simulink model "SimulinkLibrary"  (R2022b)
settings: Solver=VariableStepAuto  StartTime=0.0  StopTime=10.0  RelTol=1e-3
values from neighbouring files (symbols this model uses):
  A_w = [cosd(beta1)*sind(alfa1)  -cosd(beta2)*sind(alfa2) -cosd(beta3)*sind(alfa3) cosd(beta4)*sind(alfa4) ... (first row only)    [initfun_18072025.m]    (also in initfun_18072025_nogyro.m)
  A_wP = pinv(A_w)    [initfun_18072025.m]    (also in initfun_18072025_nogyro.m)
  C_d = 2.2    [initfun_18072025.m]    (also in initfun_18072025_nogyro.m)
  G_earth = 6.6742e-11    [initfun_18072025.m]    (also in initfun_18072025_nogyro.m)
  K = [F Z(:); Z(:)' sigma]    [Gain_matrix.m]    (also in QUEST.m = Gain_matrix(V',W',a); initfun_18072025.m = schmidt(nmax, mmax); initfun_18072025_nogyro.m = schmidt(nmax, mmax))
  m_earth = 5.9736e24    (= 5.9736e+24)    [initfun_18072025.m]    (also in initfun_18072025_nogyro.m)
  Magnetic_dipole = [0.1; 0.1;  0.1]    [initfun_18072025.m]    (also in initfun_18072025_nogyro.m)
  mmax = 3    [initfun_18072025.m]    (also in initfun_18072025_nogyro.m)
  nmax = 3    [initfun_18072025.m]    (also in initfun_18072025_nogyro.m)
  r_earth = 6371e3    (= 6371000)    [initfun_18072025.m]    (also in initfun_18072025_nogyro.m)
  RWs_Inertia = diag([9.0718e-06, 9.0718e-06, 9.0718e-06, 9.0718e-06])    [initfun_18072025.m]    (also in initfun_18072025_nogyro.m)
  RWs_Inertia_Inv = inv(RWs_Inertia)    [initfun_18072025.m]    (also in initfun_18072025_nogyro.m)
  Sat_Inertia = diag([6.295, 1.644, 5.462]*10^-1)    [initfun_18072025.m]    (also in initfun_18072025_nogyro.m)
undefined symbols (not defined in the file or in its folder): DiscIntNeverNeededParam, G, H, IAU, Sat_Aeromodel_det
libraries: matrix_library x4, vrlib x2, aerolibtransform2 x1
settings Model: Creator=LaMar  LastModifiedBy=LaMar

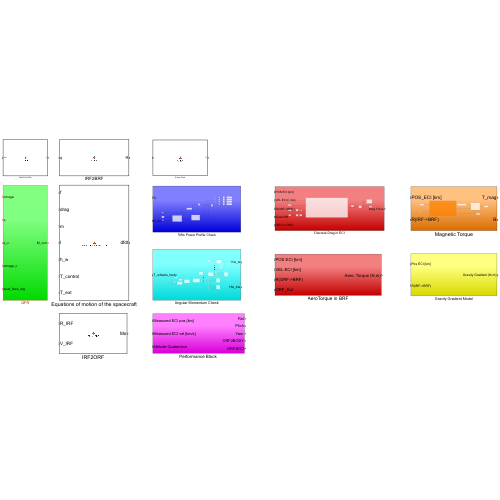
[thumbnail: Simulink's stored preview of the top-level diagram]
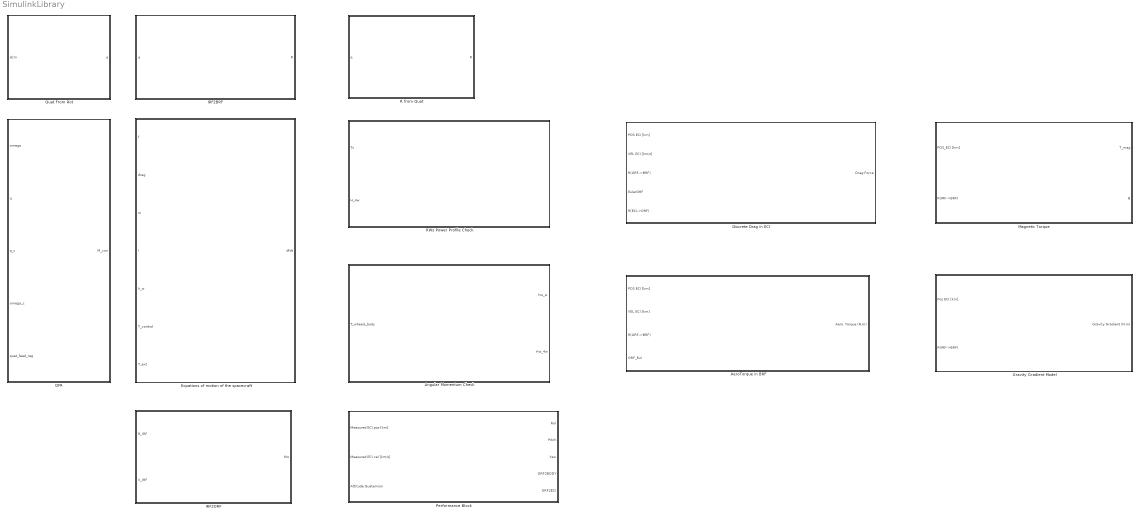
== system SimulinkLibrary ==
  AeroTorque in BRF : Subsystem
  Angular Momentum Check : Subsystem
  Discrete Drag in ECI : Subsystem
  Equations of motion of the spacecraft : MATLAB Function  TreatAsAtomicUnit=on
  Gravity Gradient Model : Subsystem
  IRF2BRF : MATLAB Function  TreatAsAtomicUnit=on
  IRF2ORF : MATLAB Function  TreatAsAtomicUnit=on
  Magnetic Torque : Subsystem
  "Performance Block " : Subsystem
  QFR : Subsystem
  Quat From Rot : MATLAB Function  TreatAsAtomicUnit=on
  R from Quat : MATLAB Function  TreatAsAtomicUnit=on
  RWs Power Profile Check : Subsystem

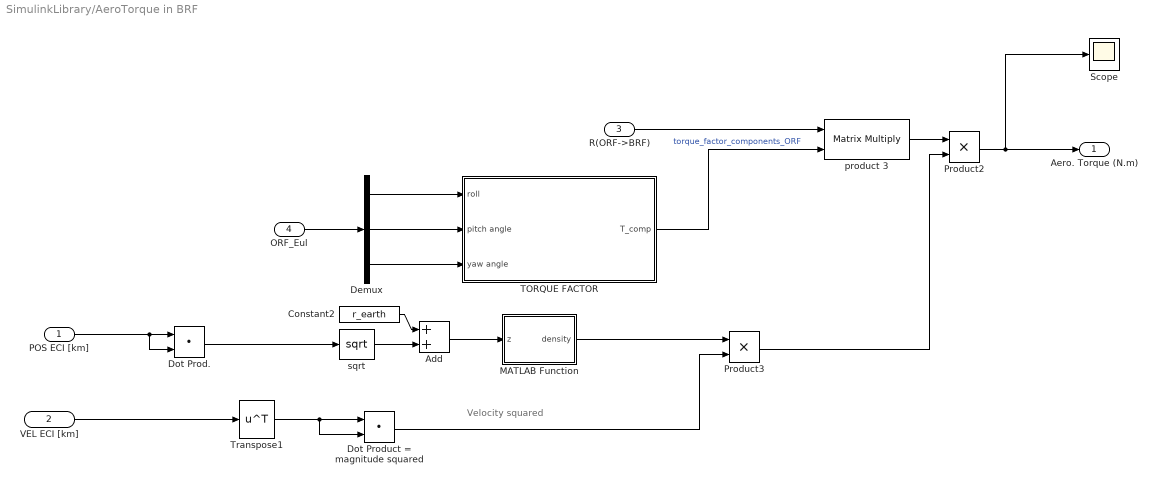
== system SimulinkLibrary/AeroTorque in BRF ==
  note: Velocity squared
  POS ECI [km] : Inport
  VEL ECI [km] : Inport  Port=2
  R(ORF->BRF) : Inport  Port=3
  ORF_Eul : Inport  Port=4
  Add : Sum
  Constant2 : Constant  Value=r_earth
  Demux : Demux  Outputs=3
  Dot Prod. : DotProduct  OutDataTypeStr=Inherit: Inherit via internal rule
  Dot Product = magnitude squared : DotProduct  OutDataTypeStr=Inherit: Inherit via internal rule
  MATLAB Function : MATLAB Function  TreatAsAtomicUnit=on
  Product2 : Product  RndMeth=Zero
  Product3 : Product  RndMeth=Zero
  Scope : Scope
  TORQUE FACTOR : Subsystem
  Transpose1 : Math  Operator=transpose  SignedPower=on
  product 3 : Product  Multiplication=Matrix(*)  RndMeth=Zero
  sqrt : Math  Operator=sqrt  SignedPower=on
  Aero. Torque (N.m) : Outport
  wires:
  sqrt/1 -> Add/2
  Add/1 -> MATLAB Function/1(z)
  Constant2/1 -> Add/1
  Demux/3 -> TORQUE FACTOR/3(yaw angle)
  Demux/2 -> TORQUE FACTOR/2(pitch angle)
  Demux/1 -> TORQUE FACTOR/1(roll)
  Product2/1 -> Aero. Torque (N.m)/1, Scope/1
  Dot Product = magnitude squared/1 -> Product3/2
  MATLAB Function/1(density) -> Product3/1
  VEL ECI [km]/1 -> Transpose1/1
  Transpose1/1 -> Dot Product = magnitude squared/1, Dot Product = magnitude squared/2
  TORQUE FACTOR/1(T_comp) -> product 3/2  "torque_factor_components_ORF"
  product 3/1 -> Product2/1
  Product3/1 -> Product2/2
  Dot Prod./1 -> sqrt/1
  POS ECI [km]/1 -> Dot Prod./2, Dot Prod./1
  R(ORF->BRF)/1 -> product 3/1
  ORF_Eul/1 -> Demux/1

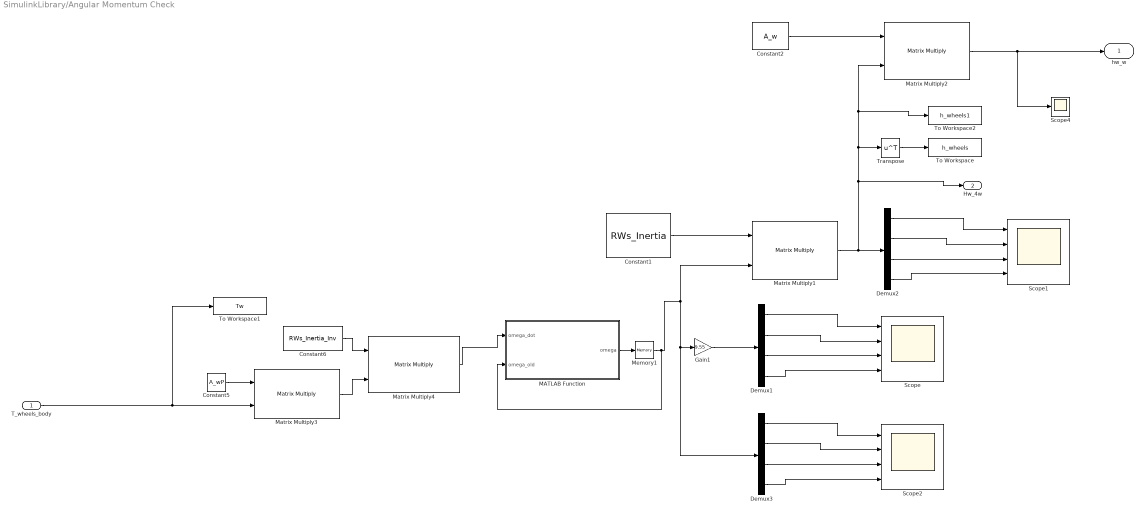
== system SimulinkLibrary/Angular Momentum Check ==
  T_wheels_body : Inport
  Constant1 : Constant  Value=RWs_Inertia
  Constant2 : Constant  Value=A_w
  Constant5 : Constant  Value=A_wP
  Constant6 : Constant  Value=RWs_Inertia_Inv
  Demux1 : Demux
  Demux2 : Demux
  Demux3 : Demux
  Gain1 : Gain  Gain=9.55
  MATLAB Function : MATLAB Function  TreatAsAtomicUnit=on
  Matrix Multiply{1..4} (4 alike) : Product  Multiplication=Matrix(*)
  Memory1 : Memory  InitialCondition=zeros(4,1)
  Scope : Scope  NumInputPorts=4
  Scope1 : Scope  NumInputPorts=4
  Scope2 : Scope  NumInputPorts=4
  Scope4 : Scope
  To Workspace : ToWorkspace  VariableName=h_wheels  SaveFormat=Structure  SampleTime=-1
      settings: Save2DSignal=2-D array (concatenate along first dimension)
  To Workspace1 : ToWorkspace  VariableName=Tw  SaveFormat=Structure With Time  SampleTime=-1
  To Workspace2 : ToWorkspace  VariableName=h_wheels1  SaveFormat=Structure  SampleTime=-1
      settings: Save2DSignal=2-D array (concatenate along first dimension)
  Transpose : Math  Operator=transpose
  hw_w : Outport
  Hw_4w : Outport  Port=2
  wires:
  Matrix Multiply1/1 -> Hw_4w/1, Transpose/1, To Workspace2/1, Matrix Multiply2/2, Demux2/1
  Constant2/1 -> Matrix Multiply2/1
  Demux1/4 -> Scope/4
  Matrix Multiply2/1 -> Scope4/1, hw_w/1
  Gain1/1 -> Demux1/1
  Demux1/3 -> Scope/3
  Demux1/2 -> Scope/2
  Demux1/1 -> Scope/1
  Constant5/1 -> Matrix Multiply3/1
  Constant1/1 -> Matrix Multiply1/1
  Demux2/3 -> Scope1/3
  Demux2/1 -> Scope1/1
  T_wheels_body/1 -> Matrix Multiply3/2, To Workspace1/1
  Demux2/4 -> Scope1/4
  Constant6/1 -> Matrix Multiply4/1
  Matrix Multiply3/1 -> Matrix Multiply4/2
  Demux2/2 -> Scope1/2
  Matrix Multiply4/1 -> MATLAB Function/1(omega_dot)
  MATLAB Function/1(omega) -> Memory1/1
  Demux3/3 -> Scope2/3
  Memory1/1 -> MATLAB Function/2(omega_old), Demux3/1, Gain1/1, Matrix Multiply1/2
  Demux3/2 -> Scope2/2
  Demux3/4 -> Scope2/4
  Demux3/1 -> Scope2/1
  Transpose/1 -> To Workspace/1

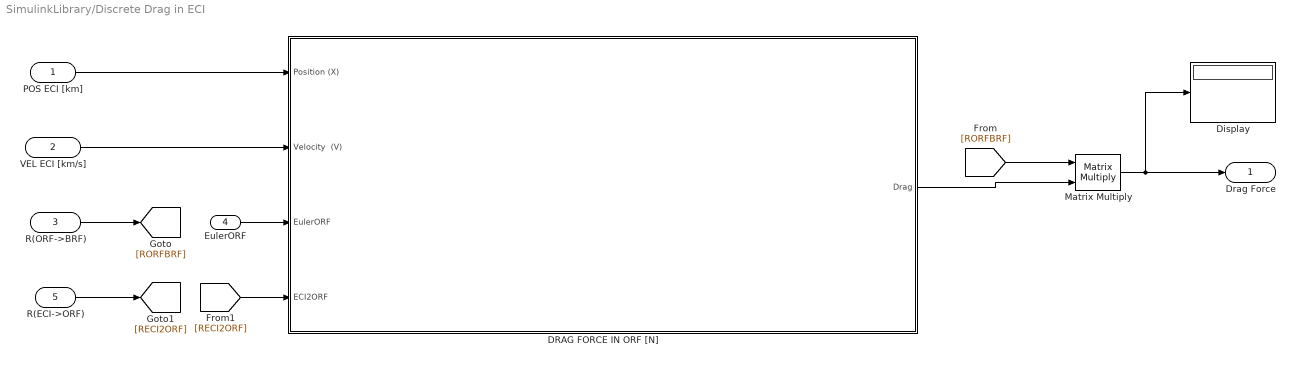
== system SimulinkLibrary/Discrete Drag in ECI ==
  POS ECI [km] : Inport
  VEL ECI [km/s] : Inport  Port=2
  R(ORF->BRF) : Inport  Port=3
  EulerORF : Inport  Port=4
  R(ECI->ORF) : Inport  Port=5
  DRAG FORCE IN ORF [N] : Subsystem
  Display : Display
  Matrix Multiply : Product  Multiplication=Matrix(*)
  Drag Force : Outport
  wires:
  R(ORF->BRF)/1 -> [RORFBRF]
  VEL ECI [km/s]/1 -> DRAG FORCE IN ORF [N]/2(Velocity  (V))
  POS ECI [km]/1 -> DRAG FORCE IN ORF [N]/1(Position (X))
  DRAG FORCE IN ORF [N]/1(Drag) -> Matrix Multiply/2
  Matrix Multiply/1 -> Display/1, Drag Force/1
  [RORFBRF] -> Matrix Multiply/1
  EulerORF/1 -> DRAG FORCE IN ORF [N]/3(EulerORF)
  [RECI2ORF] -> DRAG FORCE IN ORF [N]/4(ECI2ORF)
  R(ECI->ORF)/1 -> [RECI2ORF]

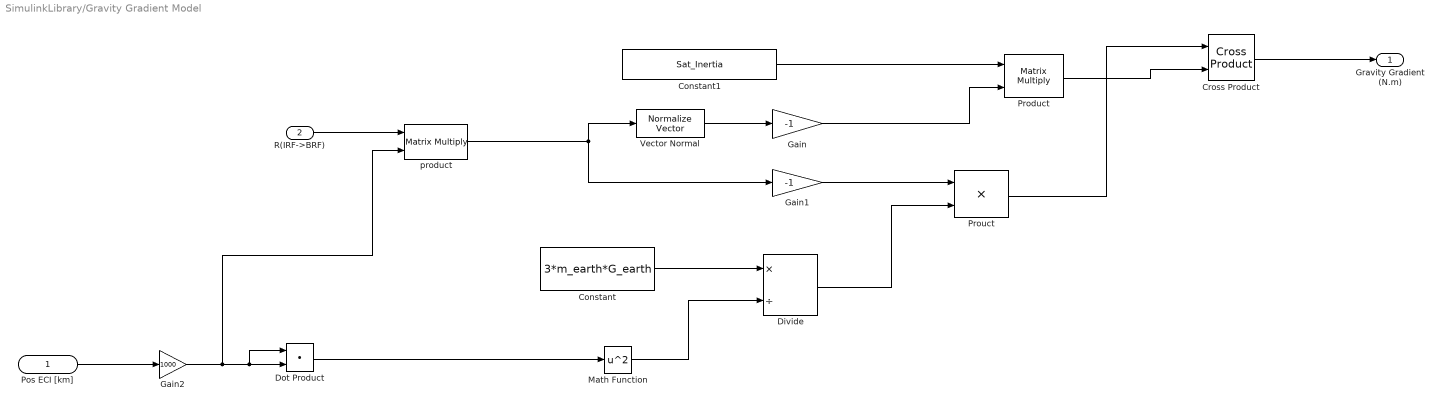
== system SimulinkLibrary/Gravity Gradient Model ==
  Pos ECI [km] : Inport
  R(IRF->BRF) : Inport  Port=2
  Constant : Constant  Value=3*m_earth*G_earth
  Constant1 : Constant  Value=Sat_Inertia
  Cross Product : matrix_library/Cross Product
  Divide : Product  Inputs=*/
  Dot Product : DotProduct  OutDataTypeStr=Inherit: Inherit via internal rule
  Gain : Gain  Gain=-1
  Gain1 : Gain  Gain=-1
  Gain2 : Gain  Gain=1000
  Math Function : Math  Operator=square  SignedPower=on
  Product : Product  Multiplication=Matrix(*)  RndMeth=Zero
  Prouct : Product  RndMeth=Zero
  Vector Normal : vrlib/Utilities/Normalize Vector  maxzero=0
  "product " : Product  Multiplication=Matrix(*)  RndMeth=Zero
  Gravity Gradient (N.m) : Outport
  wires:
  Divide/1 -> Prouct/2
  Constant/1 -> Divide/1
  Math Function/1 -> Divide/2
  Vector Normal/1 -> Gain/1
  Cross Product/1 -> Gravity Gradient (N.m)/1
  Dot Product/1 -> Math Function/1
  Product/1 -> Cross Product/2
  Constant1/1 -> Product/1
  "product "/1 -> Vector Normal/1, Gain1/1
  Gain1/1 -> Prouct/1
  Pos ECI [km]/1 -> Gain2/1
  Gain/1 -> Product/2
  Prouct/1 -> Cross Product/1
  R(IRF->BRF)/1 -> "product "/1
  Gain2/1 -> "product "/2, Dot Product/1, Dot Product/2

== system SimulinkLibrary/Magnetic Torque ==
  POS_ECI [km] : Inport
  R(IRF->BRF) : Inport  Port=2
  Cross Product : matrix_library/Cross Product
  Earth magnetc Field : Subsystem
  m : Constant  Value=Magnetic_dipole
  T_mag : Outport
  B : Outport  Port=2
  wires:
  POS_ECI [km]/1 -> Earth magnetc Field/1(R_ECI)
  Earth magnetc Field/1("BRF Earth magnetic field (T)  ") -> Cross Product/2, B/1
  m/1 -> Cross Product/1
  Cross Product/1 -> T_mag/1
  R(IRF->BRF)/1 -> Earth magnetc Field/2(R(IRF->BRF))

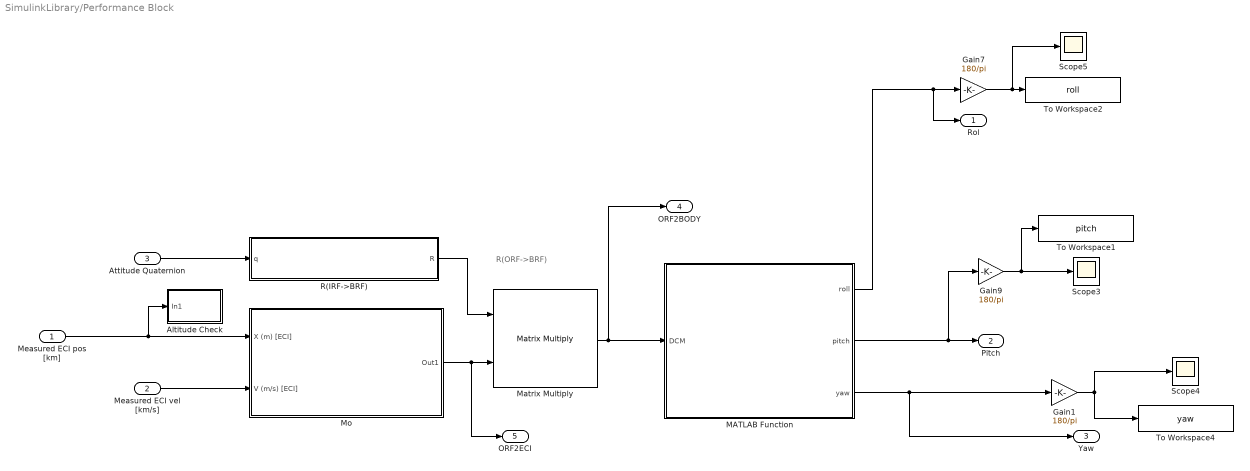
== system SimulinkLibrary/Performance Block  ==
  note: R(ORF->BRF)
  Measured ECI pos [km] : Inport
  Measured ECI vel [km/s] : Inport  Port=2
  "Attitude Quaternion " : Inport  Port=3
  Altitude Check : Subsystem
  Gain1 : Gain  Gain=180/pi
  Gain7 : Gain  Gain=180/pi
  Gain9 : Gain  Gain=180/pi
  MATLAB Function : MATLAB Function  TreatAsAtomicUnit=on
  Matrix Multiply : Product  Multiplication=Matrix(*)
  Mo : Subsystem
  R(IRF->BRF) : MATLAB Function  TreatAsAtomicUnit=on
  Scope3 : Scope
  Scope4 : Scope
  Scope5 : Scope
  To Workspace1 : ToWorkspace  VariableName=pitch  SaveFormat=Structure  SampleTime=-1
      settings: Save2DSignal=2-D array (concatenate along first dimension)
  To Workspace2 : ToWorkspace  VariableName=roll  SaveFormat=Structure  SampleTime=-1
      settings: Save2DSignal=2-D array (concatenate along first dimension)
  To Workspace4 : ToWorkspace  VariableName=yaw  SaveFormat=Structure  SampleTime=-1
      settings: Save2DSignal=2-D array (concatenate along first dimension)
  Rol : Outport
  Pitch : Outport  Port=2
  "Yaw " : Outport  Port=3
  ORF2BODY : Outport  Port=4
  ORF2ECI : Outport  Port=5
  wires:
  MATLAB Function/3(yaw) -> "Yaw "/1, Gain1/1
  MATLAB Function/1(roll) -> Gain7/1, Rol/1
  "Attitude Quaternion "/1 -> R(IRF->BRF)/1(q)
  Measured ECI vel [km/s]/1 -> Mo/2(V (m/s) [ECI])
  Gain1/1 -> Scope4/1, To Workspace4/1
  MATLAB Function/2(pitch) -> Pitch/1, Gain9/1
  Matrix Multiply/1 -> ORF2BODY/1, MATLAB Function/1(DCM)
  Gain7/1 -> To Workspace2/1, Scope5/1
  Mo/1(Out1) -> ORF2ECI/1, Matrix Multiply/2
  Gain9/1 -> To Workspace1/1, Scope3/1
  R(IRF->BRF)/1(R) -> Matrix Multiply/1
  Measured ECI pos [km]/1 -> Mo/1(X (m) [ECI]), Altitude Check/1(In1)

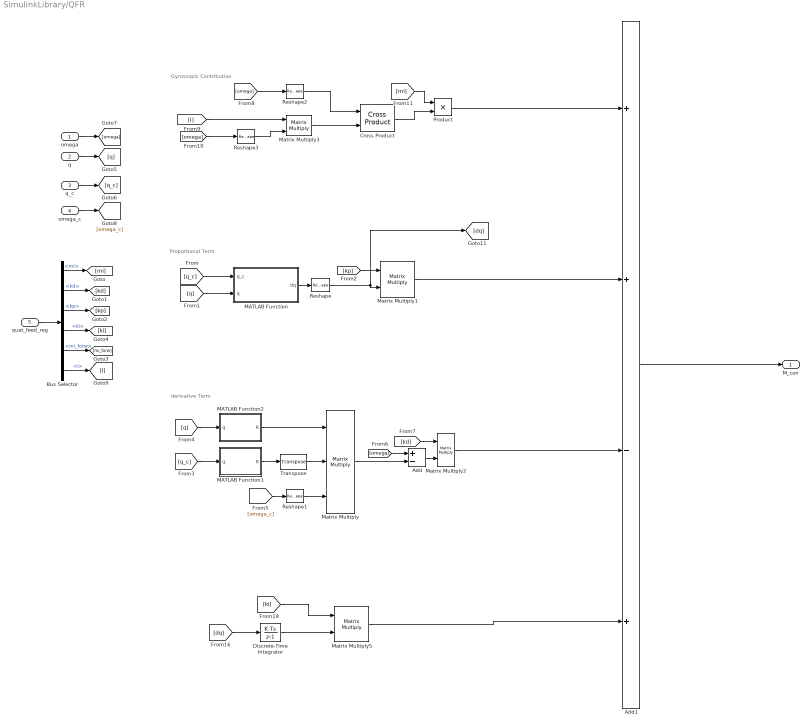
== system SimulinkLibrary/QFR ==
  note: Gyroscopic Contribution
  note: derivative Term
  note: Proportional Term
  omega : Inport
  q : Inport  Port=2
  q_c : Inport  Port=3
  omega_c : Inport  Port=4
  quat_feed_reg : Inport  Port=5
  Add : Sum  Inputs=+-
  Add1 : Sum  Inputs=++-+
  Bus Selector : BusSelector  OutputSignals=mi,kd,kp,ki,mi_forw,I
  Cross Product : matrix_library/Cross Product
  Discrete-Time Integrator : DiscreteIntegrator  InitialCondition=zeros(3,1)  SampleTime=0.5  ICPrevOutput=DiscIntNeverNeededParam  ICPrevScaledInput=DiscIntNeverNeededParam
  MATLAB Function : MATLAB Function  TreatAsAtomicUnit=on
  MATLAB Function1 : MATLAB Function  TreatAsAtomicUnit=on
  MATLAB Function2 : MATLAB Function  TreatAsAtomicUnit=on
  Matrix Multiply : Product  Inputs=3  Multiplication=Matrix(*)
  Matrix Multiply{1..3,5} (4 alike) : Product  Multiplication=Matrix(*)
  Product : Product
  Reshape{,1..3} (4 alike) : Reshape  OutputDimensionality=Column vector (2-D)
  Transpose : matrix_library/Transpose
  M_con : Outport
  wires:
  quat_feed_reg/1 -> Bus Selector/1
  Bus Selector/1 -> [mi]  "<mi>"
  Bus Selector/2 -> [kd]  "<kd>"
  Bus Selector/3 -> [kp]  "<kp>"
  Bus Selector/4 -> [ki]  "<ki>"
  Bus Selector/5 -> [mi_forw]  "<mi_forw>"
  q/1 -> [q]
  q_c/1 -> [q_c]
  omega/1 -> [omega]
  omega_c/1 -> [omega_c]
  [q_c] -> MATLAB Function/1(q_c)
  [q] -> MATLAB Function/2(q)
  MATLAB Function/1(dq) -> Reshape/1
  [q_c] -> MATLAB Function1/1(q)
  MATLAB Function1/1(R) -> Transpose/1
  Transpose/1 -> Matrix Multiply/2
  [q] -> MATLAB Function2/1(q)
  MATLAB Function2/1(R) -> Matrix Multiply/1
  [omega_c] -> Reshape1/1
  Reshape1/1 -> Matrix Multiply/3
  Matrix Multiply/1 -> Add/2
  [omega] -> Add/1
  [kp] -> Matrix Multiply1/1
  Reshape/1 -> [dq], Matrix Multiply1/2
  Add/1 -> Matrix Multiply2/2
  [kd] -> Matrix Multiply2/1
  Bus Selector/6 -> [I]  "<I>"
  [omega] -> Reshape2/1
  Reshape2/1 -> Cross Product/1
  [omega] -> Reshape3/1
  [I] -> Matrix Multiply3/1
  Reshape3/1 -> Matrix Multiply3/2
  Matrix Multiply3/1 -> Cross Product/2
  Cross Product/1 -> Product/2
  [mi] -> Product/1
  Product/1 -> Add1/1
  Matrix Multiply1/1 -> Add1/2
  Matrix Multiply2/1 -> Add1/3
  Add1/1 -> M_con/1
  [dq] -> Discrete-Time Integrator/1
  Discrete-Time Integrator/1 -> Matrix Multiply5/2
  [ki] -> Matrix Multiply5/1
  Matrix Multiply5/1 -> Add1/4

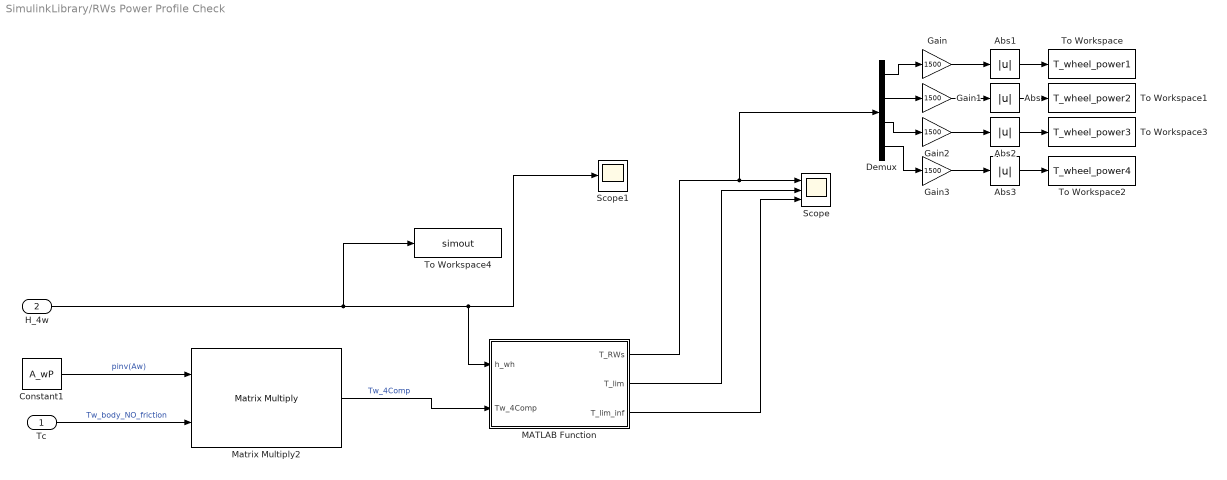
== system SimulinkLibrary/RWs Power Profile Check ==
  Tc : Inport
  H_4w : Inport  Port=2
  Abs{,1..3} (4 alike) : Abs  SaturateOnIntegerOverflow=off
  Constant1 : Constant  Value=A_wP
  Demux : Demux
  Gain{,1..3} (4 alike) : Gain  Gain=1500
  MATLAB Function : MATLAB Function  TreatAsAtomicUnit=on
  Matrix Multiply2 : Product  Multiplication=Matrix(*)
  Scope : Scope  NumInputPorts=3
  Scope1 : Scope
  To Workspace : ToWorkspace  VariableName=T_wheel_power1  SaveFormat=Timeseries  SampleTime=-1
  To Workspace1 : ToWorkspace  VariableName=T_wheel_power2  SaveFormat=Timeseries  SampleTime=-1
  To Workspace2 : ToWorkspace  VariableName=T_wheel_power4  SaveFormat=Timeseries  SampleTime=-1
  To Workspace3 : ToWorkspace  VariableName=T_wheel_power3  SaveFormat=Timeseries  SampleTime=-1
  To Workspace4 : ToWorkspace  VariableName=simout  SaveFormat=Timeseries  SampleTime=-1
  wires:
  Constant1/1 -> Matrix Multiply2/1  "pinv(Aw)"
  Matrix Multiply2/1 -> MATLAB Function/2(Tw_4Comp)  "Tw_4Comp"
  Tc/1 -> Matrix Multiply2/2  "Tw_body_NO_friction"
  MATLAB Function/1(T_RWs) -> Demux/1, Scope/1
  H_4w/1 -> To Workspace4/1, Scope1/1, MATLAB Function/1(h_wh)
  MATLAB Function/3(T_lim_inf) -> Scope/3
  Demux/2 -> Gain1/1
  Demux/1 -> Gain/1
  Demux/3 -> Gain2/1
  Demux/4 -> Gain3/1
  Gain2/1 -> Abs2/1
  Gain1/1 -> Abs/1
  Gain/1 -> Abs1/1
  Gain3/1 -> Abs3/1
  MATLAB Function/2(T_lim) -> Scope/2
  Abs1/1 -> To Workspace/1
  Abs/1 -> To Workspace1/1
  Abs3/1 -> To Workspace2/1
  Abs2/1 -> To Workspace3/1

== system SimulinkLibrary/AeroTorque in BRF/TORQUE FACTOR ==
  roll : Inport
  pitch angle : Inport  Port=2
  yaw angle : Inport  Port=3
  MATLAB Function : MATLAB Function  TreatAsAtomicUnit=on
  Merge : Merge
  Subsystem : Subsystem
  Subsystem1 : Subsystem
  T_comp : Outport
  wires:
  Subsystem1/1(T_components) -> Merge/2
  Merge/1 -> T_comp/1
  Subsystem/1(T_components) -> Merge/1
  MATLAB Function/2(out2) -> Subsystem1/Enable
  MATLAB Function/1(out1) -> Subsystem/Enable
  yaw angle/1 -> MATLAB Function/3(yaw_angle), Subsystem/3(yaw angle), Subsystem1/3(yaw angle)
  pitch angle/1 -> MATLAB Function/2(pitch_angle), Subsystem/2(pitch angle), Subsystem1/2(pitch angle)
  roll/1 -> MATLAB Function/1(roll_angle), Subsystem/1(roll), Subsystem1/1(roll)

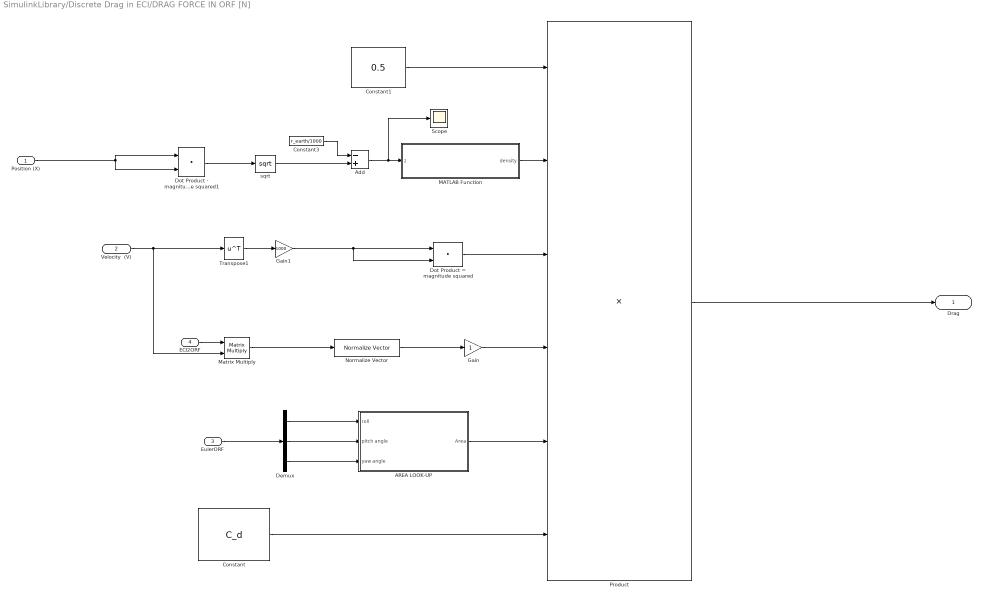
== system SimulinkLibrary/Discrete Drag in ECI/DRAG FORCE IN ORF [N] ==
  Position (X) : Inport
  Velocity  (V) : Inport  Port=2
  EulerORF : Inport  Port=3
  ECI2ORF : Inport  Port=4
  AREA LOOK-UP : Subsystem
  Add : Sum  Inputs=-+
  Constant : Constant  Value=C_d
  Constant1 : Constant  Value=0.5
  Constant3 : Constant  Value=r_earth/1000
  Demux : Demux  Outputs=3
  Dot Product - magnitude squared1 : DotProduct  OutDataTypeStr=Inherit: Inherit via internal rule
  Dot Product = magnitude squared : DotProduct  OutDataTypeStr=Inherit: Inherit via internal rule
  Gain : Gain
  Gain1 : Gain  Gain=1000
  MATLAB Function : MATLAB Function  TreatAsAtomicUnit=on
  Matrix Multiply : Product  Multiplication=Matrix(*)
  Normalize Vector : vrlib/Utilities/Normalize Vector  maxzero=0
  Product : Product  Inputs=6
  Scope : Scope
  Transpose1 : Math  Operator=transpose  SignedPower=on
  sqrt : Math  Operator=sqrt  SignedPower=on
  Drag : Outport
  wires:
  sqrt/1 -> Add/2
  Add/1 -> Scope/1, MATLAB Function/1(z)
  MATLAB Function/1(density) -> Product/2
  Constant3/1 -> Add/1
  Demux/3 -> AREA LOOK-UP/3(yaw angle)
  Demux/2 -> AREA LOOK-UP/2(pitch angle)
  Demux/1 -> AREA LOOK-UP/1(roll)
  Product/1 -> Drag/1
  Dot Product = magnitude squared/1 -> Product/3
  Gain/1 -> Product/4
  Normalize Vector/1 -> Gain/1
  Constant1/1 -> Product/1
  AREA LOOK-UP/1(Area) -> Product/5
  Constant/1 -> Product/6
  Velocity  (V)/1 -> Matrix Multiply/2, Transpose1/1
  Transpose1/1 -> Gain1/1
  Position (X)/1 -> Dot Product - magnitude squared1/1, Dot Product - magnitude squared1/2
  Dot Product - magnitude squared1/1 -> sqrt/1
  EulerORF/1 -> Demux/1
  ECI2ORF/1 -> Matrix Multiply/1
  Matrix Multiply/1 -> Normalize Vector/1
  Gain1/1 -> Dot Product = magnitude squared/1, Dot Product = magnitude squared/2

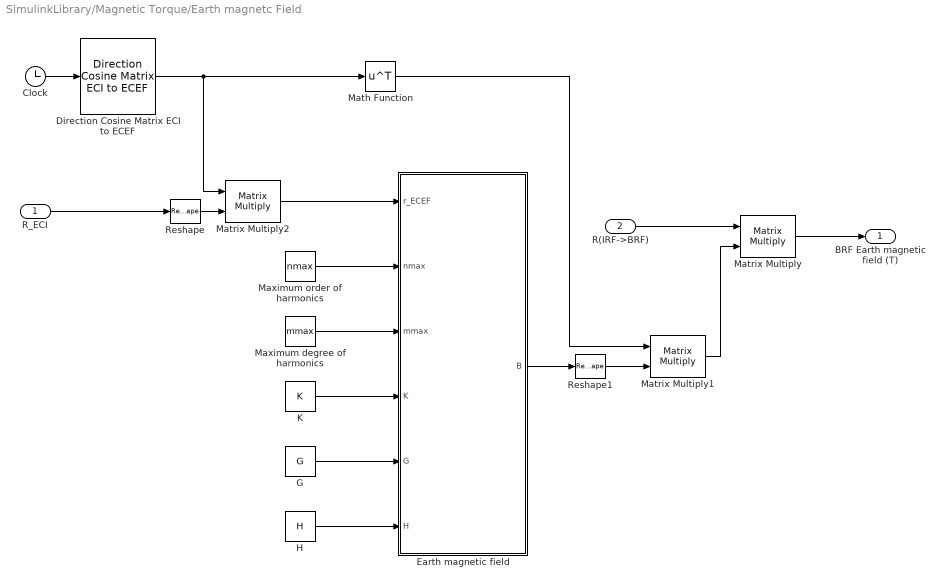
== system SimulinkLibrary/Magnetic Torque/Earth magnetc Field ==
  R_ECI : Inport
  R(IRF->BRF) : Inport  Port=2
  Clock : Clock
  Direction Cosine Matrix ECI to ECEF : aerolibtransform2/Direction Cosine Matrix ECI to ECEF  red=IAU-2000/2006  year=2020  month=December  day=1  hour=10  min=0  sec=0  deltaT=Sec  errorflag=Error  extraparamflag=off
      settings: AttributesFormatString=%<red>
  "Earth magnetic field " : MATLAB Function  TreatAsAtomicUnit=on
  G : Constant  Value=G  VectorParams1D=off
  H : Constant  Value=H  VectorParams1D=off
  K : Constant  Value=K  VectorParams1D=off
  Math Function : Math  Operator=transpose  SignedPower=on
  Matrix Multiply : Product  Multiplication=Matrix(*)
  Matrix Multiply1 : Product  Multiplication=Matrix(*)
  Matrix Multiply2 : Product  Multiplication=Matrix(*)
  "Maximum degree of harmonics " : Constant  Value=mmax
  "Maximum order of harmonics " : Constant  Value=nmax
  Reshape : Reshape  OutputDimensionality=Column vector (2-D)
  Reshape1 : Reshape  OutputDimensionality=Column vector (2-D)
  "BRF Earth magnetic field (T)  " : Outport
  wires:
  R(IRF->BRF)/1 -> Matrix Multiply/1
  Matrix Multiply/1 -> "BRF Earth magnetic field (T)  "/1
  Math Function/1 -> Matrix Multiply1/1
  "Earth magnetic field "/1(B) -> Reshape1/1
  Matrix Multiply2/1 -> "Earth magnetic field "/1(r_ECEF)
  Direction Cosine Matrix ECI to ECEF/1 -> Matrix Multiply2/1, Math Function/1
  Matrix Multiply1/1 -> Matrix Multiply/2
  Clock/1 -> Direction Cosine Matrix ECI to ECEF/1
  H/1 -> "Earth magnetic field "/6(H)
  "Maximum order of harmonics "/1 -> "Earth magnetic field "/2(nmax)
  "Maximum degree of harmonics "/1 -> "Earth magnetic field "/3(mmax)
  G/1 -> "Earth magnetic field "/5(G)
  K/1 -> "Earth magnetic field "/4(K)
  Reshape/1 -> Matrix Multiply2/2
  Reshape1/1 -> Matrix Multiply1/2
  R_ECI/1 -> Reshape/1

== system SimulinkLibrary/Performance Block /Altitude Check ==
  In1 : Inport
  Constant : Constant  Value=6378
  Dot Product : DotProduct  OutDataTypeStr=Inherit: Inherit via internal rule
  Scope : Scope
  Square Root : Sqrt
  Subtract : Sum  Inputs=+-
  wires:
  In1/1 -> Dot Product/1, Dot Product/2
  Constant/1 -> Subtract/2
  Square Root/1 -> Subtract/1
  Dot Product/1 -> Square Root/1
  Subtract/1 -> Scope/1

== system SimulinkLibrary/Performance Block /Mo ==
  X (m) [ECI] : Inport
  V (m/s) [ECI] : Inport  Port=2
  MATLAB Function : MATLAB Function  TreatAsAtomicUnit=on
  Transpose : Math  Operator=transpose
  Out1 : Outport
  wires:
  Transpose/1 -> Out1/1
  MATLAB Function/1(Mo) -> Transpose/1
  X (m) [ECI]/1 -> MATLAB Function/1(X)
  V (m/s) [ECI]/1 -> MATLAB Function/2(V)

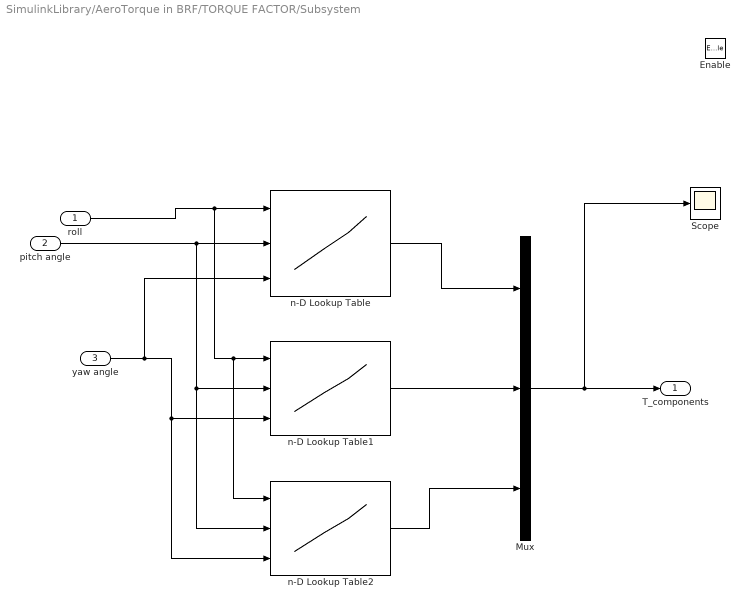
== system SimulinkLibrary/AeroTorque in BRF/TORQUE FACTOR/Subsystem ==
  roll : Inport
  pitch angle : Inport  Port=2
  yaw angle : Inport  Port=3
  Enable : EnablePort
  Mux : Mux  Inputs=3
  Scope : Scope
  n-D Lookup Table : Lookup_n-D  NumberOfTableDimensions=3  BreakpointsForDimension1=Sat_Aeromodel_det.roll  BreakpointsForDimension2=Sat_Aeromodel_det.pitch  BreakpointsForDimension3=Sat_Aeromodel_det.yaw  Table=Sat_Aeromodel_det.xComp  InterpMethod=Cubic spline  ExtrapMethod=Cubic spline  InternalRulePriority=Speed  RndMeth=Simplest
      settings: InputPortMap=u0,u1,u2
  n-D Lookup Table1 : Lookup_n-D  NumberOfTableDimensions=3  BreakpointsForDimension1=Sat_Aeromodel_det.roll  BreakpointsForDimension2=Sat_Aeromodel_det.pitch  BreakpointsForDimension3=Sat_Aeromodel_det.yaw  Table=Sat_Aeromodel_det.yComp  InterpMethod=Cubic spline  ExtrapMethod=Cubic spline  InternalRulePriority=Speed  RndMeth=Simplest
      settings: InputPortMap=u0,u1,u2
  n-D Lookup Table2 : Lookup_n-D  NumberOfTableDimensions=3  BreakpointsForDimension1=Sat_Aeromodel_det.roll  BreakpointsForDimension2=Sat_Aeromodel_det.pitch  BreakpointsForDimension3=Sat_Aeromodel_det.yaw  Table=Sat_Aeromodel_det.zComp  InterpMethod=Cubic spline  ExtrapMethod=Cubic spline  InternalRulePriority=Speed  RndMeth=Simplest
      settings: InputPortMap=u0,u1,u2
  T_components : Outport
  wires:
  yaw angle/1 -> n-D Lookup Table/3, n-D Lookup Table1/3, n-D Lookup Table2/3
  pitch angle/1 -> n-D Lookup Table/2, n-D Lookup Table1/2, n-D Lookup Table2/2
  roll/1 -> n-D Lookup Table/1, n-D Lookup Table1/1, n-D Lookup Table2/1
  n-D Lookup Table2/1 -> Mux/3
  Mux/1 -> T_components/1, Scope/1
  n-D Lookup Table/1 -> Mux/1
  n-D Lookup Table1/1 -> Mux/2

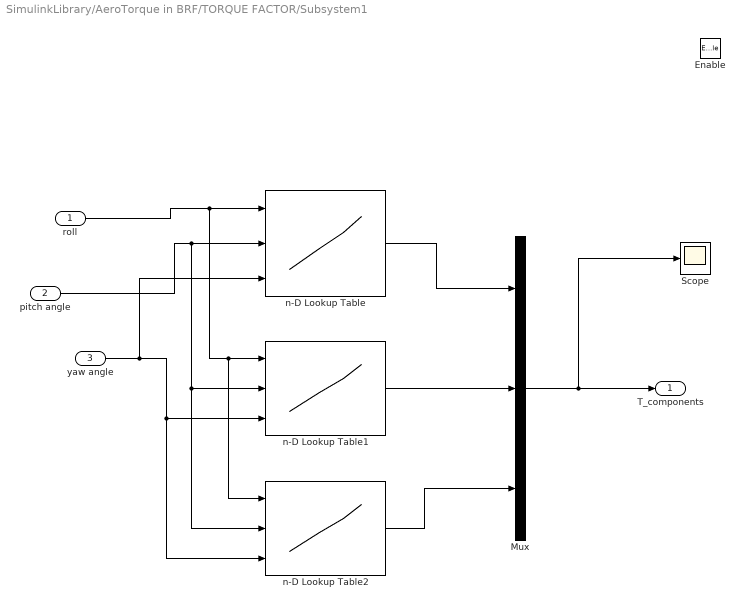
== system SimulinkLibrary/AeroTorque in BRF/TORQUE FACTOR/Subsystem1 ==
  roll : Inport
  pitch angle : Inport  Port=2
  yaw angle : Inport  Port=3
  Enable : EnablePort
  Mux : Mux  Inputs=3
  Scope : Scope
  n-D Lookup Table : Lookup_n-D  NumberOfTableDimensions=3  BreakpointsForDimension1=Sat_Aeromodel_det.roll  BreakpointsForDimension2=Sat_Aeromodel_det.pitch  BreakpointsForDimension3=Sat_Aeromodel_det.yaw  Table=Sat_Aeromodel_det.xComp  InterpMethod=Cubic spline  ExtrapMethod=Cubic spline  InternalRulePriority=Speed  RndMeth=Simplest
      settings: InputPortMap=u0,u1,u2
  n-D Lookup Table1 : Lookup_n-D  NumberOfTableDimensions=3  BreakpointsForDimension1=Sat_Aeromodel_det.roll  BreakpointsForDimension2=Sat_Aeromodel_det.pitch  BreakpointsForDimension3=Sat_Aeromodel_det.yaw  Table=Sat_Aeromodel_det.yComp  InterpMethod=Cubic spline  ExtrapMethod=Cubic spline  InternalRulePriority=Speed  RndMeth=Simplest
      settings: InputPortMap=u0,u1,u2
  n-D Lookup Table2 : Lookup_n-D  NumberOfTableDimensions=3  BreakpointsForDimension1=Sat_Aeromodel_det.roll  BreakpointsForDimension2=Sat_Aeromodel_det.pitch  BreakpointsForDimension3=Sat_Aeromodel_det.yaw  Table=Sat_Aeromodel_det.zComp  InterpMethod=Cubic spline  ExtrapMethod=Cubic spline  InternalRulePriority=Speed  RndMeth=Simplest
      settings: InputPortMap=u0,u1,u2
  T_components : Outport
  wires:
  yaw angle/1 -> n-D Lookup Table/3, n-D Lookup Table1/3, n-D Lookup Table2/3
  pitch angle/1 -> n-D Lookup Table/2, n-D Lookup Table1/2, n-D Lookup Table2/2
  roll/1 -> n-D Lookup Table/1, n-D Lookup Table1/1, n-D Lookup Table2/1
  n-D Lookup Table2/1 -> Mux/3
  Mux/1 -> T_components/1, Scope/1
  n-D Lookup Table/1 -> Mux/1
  n-D Lookup Table1/1 -> Mux/2

== system SimulinkLibrary/Discrete Drag in ECI/DRAG FORCE IN ORF [N]/AREA LOOK-UP ==
  roll : Inport
  pitch angle : Inport  Port=2
  yaw angle : Inport  Port=3
  MATLAB Function : MATLAB Function  TreatAsAtomicUnit=on
  Merge : Merge
  Subsystem : Subsystem
  Subsystem1 : Subsystem
  Area : Outport
  wires:
  Merge/1 -> Area/1
  Subsystem1/1(Area) -> Merge/2
  Subsystem/1(Area) -> Merge/1
  MATLAB Function/2(out2) -> Subsystem1/Enable
  MATLAB Function/1(out1) -> Subsystem/Enable
  yaw angle/1 -> MATLAB Function/3(yaw_angle), Subsystem/3(yaw angle), Subsystem1/3(yaw angle)
  pitch angle/1 -> MATLAB Function/2(pitch_angle), Subsystem/2(pitch angle), Subsystem1/2(pitch angle)
  roll/1 -> MATLAB Function/1(roll_angle), Subsystem/1(roll), Subsystem1/1(roll)

== system SimulinkLibrary/Discrete Drag in ECI/DRAG FORCE IN ORF [N]/AREA LOOK-UP/Subsystem ==
  roll : Inport
  pitch angle : Inport  Port=2
  yaw angle : Inport  Port=3
  Enable : EnablePort
  n-D Lookup Table2 : Lookup_n-D  NumberOfTableDimensions=3  BreakpointsForDimension1=Sat_Aeromodel_det.roll  BreakpointsForDimension2=Sat_Aeromodel_det.pitch  BreakpointsForDimension3=Sat_Aeromodel_det.yaw  Table=Sat_Aeromodel_det.Area  InterpMethod=Cubic spline  ExtrapMethod=Cubic spline  InternalRulePriority=Speed  RndMeth=Simplest
      settings: InputPortMap=u0,u1,u2
  Area : Outport
  wires:
  pitch angle/1 -> n-D Lookup Table2/2
  roll/1 -> n-D Lookup Table2/1
  yaw angle/1 -> n-D Lookup Table2/3
  n-D Lookup Table2/1 -> Area/1

== system SimulinkLibrary/Discrete Drag in ECI/DRAG FORCE IN ORF [N]/AREA LOOK-UP/Subsystem1 ==
  roll : Inport
  pitch angle : Inport  Port=2
  yaw angle : Inport  Port=3
  Enable : EnablePort
  n-D Lookup Table2 : Lookup_n-D  NumberOfTableDimensions=3  BreakpointsForDimension1=Sat_Aeromodel_det.roll  BreakpointsForDimension2=Sat_Aeromodel_det.pitch  BreakpointsForDimension3=Sat_Aeromodel_det.yaw  Table=Sat_Aeromodel_det.Area  InterpMethod=Cubic spline  ExtrapMethod=Cubic spline  InternalRulePriority=Speed  RndMeth=Simplest
      settings: InputPortMap=u0,u1,u2
  Area : Outport
  wires:
  pitch angle/1 -> n-D Lookup Table2/2
  roll/1 -> n-D Lookup Table2/1
  yaw angle/1 -> n-D Lookup Table2/3
  n-D Lookup Table2/1 -> Area/1

== matlab function SimulinkLibrary/QFR/MATLAB Function ==
  data: q_c input; dq output; q input
function dq  = qmultiply(q_c,q)
%#codegen
%% Quaternion multiplication
% qs = ps*rs - pv'*rv
% qv = ps*rv + rs*pv - pv x rv
%r(1:3) = -r(1:3);
%% INPUT 
% p: vector 4x1
% r: vector 4x1

%% OUTPUT
% q: vector 4x1

% N.B. The first component of the quaternion is the scalar part
q(1:3) = -q(1:3);
% q(4) = p(4)*r(4) - p(1:3)'*r(1:3);
% q(1:3) = p(4)*r(1:3) + r(4)*p(1:3) - cross(p(1:3),r(1:3));
dqs=zeros(4,1);
dqs(1:3,1) = q_c(4)*q(1:3)+q(4)*q_c(1:3)-cross(q_c(1:3),q(1:3));
dqs(4,1) = q_c(4)*q(4)-q_c(1:3)'*q(1:3);
dq = sign(dqs(4))*dqs(1:3);
appo = q(1:4);
end

== matlab function SimulinkLibrary/QFR/MATLAB Function1 ==
  data: q input; R output
function R = R_by_q(q)

%% Description 
% This block provides the rotation matrix corresponding to the quaternion
% in input. THE SCALAR LAST CONVENTION IS USED FOR THE QUATERNION

%% INPUT 
% q -> 4x1 array (quaternion)
%% OUTPUT 
% R -> 3x3 matrix (rotation matrix)
q0 = q(4); 
q1 = q(1);
q2 = q(2);
q3 = q(3);

R = [q0^2+q1^2-q2^2-q3^2 2*q1*q2+2*q0*q3 2*q1*q3-2*q0*q2;
    2*q1*q2-2*q0*q3 q0^2-q1^2+q2^2-q3^2 2*q2*q3+2*q0*q1;
    2*q1*q3+2*q0*q2 2*q2*q3-2*q0*q1 q0^2-q1^2-q2^2+q3^2];
end

== matlab function SimulinkLibrary/AeroTorque in BRF/TORQUE FACTOR/MATLAB Function ==
  data: roll_angle input; out1 output; pitch_angle input; yaw_angle input; out2 output
function [out1, out2]= aero_selection(roll_angle, pitch_angle, yaw_angle)


if abs(roll_angle)>0.2618
    out1=1;
    out2=0;

else if abs(pitch_angle)>0.2618

        out1=1;
        out2=0;
else if abs(yaw_angle)>0.2618

        out1=1;
        out2=0;
else
    out1=0;
    out2=1;
end
end
end
end

== matlab function SimulinkLibrary/QFR/MATLAB Function2 ==
  data: q input; R output
function R = R_by_q(q)

%% Description 
% This block provides the rotation matrix corresponding to the quaternion
% in input. THE SCALAR LAST CONVENTION IS USED FOR THE QUATERNION

%% INPUT 
% q -> 4x1 array (quaternion)
%% OUTPUT 
% R -> 3x3 matrix (rotation matrix)
q0 = q(4); 
q1 = q(1);
q2 = q(2);
q3 = q(3);

R = [q0^2+q1^2-q2^2-q3^2 2*q1*q2+2*q0*q3 2*q1*q3-2*q0*q2;
    2*q1*q2-2*q0*q3 q0^2-q1^2+q2^2-q3^2 2*q2*q3+2*q0*q1;
    2*q1*q3+2*q0*q2 2*q2*q3-2*q0*q1 q0^2-q1^2-q2^2+q3^2];
end

== matlab function SimulinkLibrary/Discrete Drag in ECI/DRAG FORCE IN ORF [N]/AREA LOOK-UP/MATLAB Function ==
  data: roll_angle input; out1 output; pitch_angle input; yaw_angle input; out2 output
function [out1, out2]= aero_selection(roll_angle, pitch_angle, yaw_angle)


if abs(roll_angle)>0.2618
    out1=1;
    out2=0;

else if abs(pitch_angle)>0.2618

        out1=1;
        out2=0;
else if abs(yaw_angle)>0.2618

        out1=1;
        out2=0;
else
    out1=0;
    out2=1;
end
end
end
end

== matlab function SimulinkLibrary/R from Quat ==
  data: q input; R output
function R = R_by_q(q)

%% Description 
% This block provides the rotation matrix corresponding to the quaternion
% in input. THE SCALAR LAST CONVENTION IS USED FOR THE QUATERNION

%% INPUT 
% q -> 4x1 array (quaternion)
%% OUTPUT 
% R -> 3x3 matrix (rotation matrix)
q0 = q(4); 
q1 = q(1);
q2 = q(2);
q3 = q(3);

R = [q0^2+q1^2-q2^2-q3^2 2*q1*q2+2*q0*q3 2*q1*q3-2*q0*q2;
    2*q1*q2-2*q0*q3 q0^2-q1^2+q2^2-q3^2 2*q2*q3+2*q0*q1;
    2*q1*q3+2*q0*q2 2*q2*q3-2*q0*q1 q0^2-q1^2-q2^2+q3^2];
end

== matlab function SimulinkLibrary/Quat From Rot ==
  data: dcm input; q output
function q = q_by_R(dcm)
%% Description 
% This block provides the quaternion corresponding to the rotation matrix 
% in input. THE SCALAR LAST CONVENTION IS USED FOR THE QUATERNION. 
%% INPUT 
% R -> 3x3 matrix (rotation matrix)
%% OUTPUT 
% q -> 4x1 array (quaternion)
q = zeros(4,1);
tr = trace(dcm);
 if (tr > 0)
        sqtrp1 = sqrt( tr + 1.0 );
        q(4) = 0.5*sqtrp1; 
        q(1) = (dcm(2, 3) - dcm(3, 2))/(2.0*sqtrp1);
        q(2) = (dcm(3, 1) - dcm(1, 3))/(2.0*sqtrp1); 
        q(3) = (dcm(1, 2) - dcm(2, 1))/(2.0*sqtrp1); 
    else
        d = diag(dcm(:,:));
        if ((d(2) > d(1)) && (d(2) > d(3)))
            % max value at dcm(2,2,i)
            sqdip1 = sqrt(d(2) - d(1) - d(3) + 1.0 );
            
            q(2) = 0.5*sqdip1; 
            
            if ( sqdip1 ~= 0 )
                sqdip1 = 0.5/sqdip1;
            end
            
            q(4) = (dcm(3, 1) - dcm(1, 3))*sqdip1; 
            q(1) = (dcm(1, 2) + dcm(2, 1))*sqdip1; 
            q(3) = (dcm(2, 3) + dcm(3, 2))*sqdip1; 
        elseif (d(3) > d(1))
            % max value at dcm(3,3,i)
            sqdip1 = sqrt(d(3) - d(1) - d(2) + 1.0 );
            
            q(3) = 0.5*sqdip1; 
            
            if ( sqdip1 ~= 0 )
                sqdip1 = 0.5/sqdip1;
            end
            
            q(4) = (dcm(1, 2) - dcm(2, 1))*sqdip1;
            q(1) = (dcm(3, 1) + dcm(1, 3))*sqdip1; 
            q(2) = (dcm(2, 3) + dcm(3, 2))*sqdip1; 
        else
            % max value at dcm(1,1,i)
            sqdip1 = sqrt(d(1) - d(2) - d(3) + 1.0 );
            
            q(1) = 0.5*sqdip1; 
            
            if ( sqdip1 ~= 0 )
                sqdip1 = 0.5/sqdip1;
            end
            
            q(4) = (dcm(2, 3) - dcm(3, 2))*sqdip1; 
            q(2) = (dcm(1, 2) + dcm(2, 1))*sqdip1; 
            q(3) = (dcm(3, 1) + dcm(1, 3))*sqdip1; 
        end
 end 

end

== matlab function SimulinkLibrary/Angular Momentum Check/MATLAB Function ==
  data: omega_dot input; omega output; omega_old input
function omega = omega_new(omega_dot, omega_old)
t=1;
omega=omega_dot+omega_old;

end

== matlab function SimulinkLibrary/Performance Block /R(IRF->BRF) ==
  data: q input; R output
function R = R_by_q(q)

%% Description 
% This block provides the rotation matrix corresponding to the quaternion
% in input. THE SCALAR LAST CONVENTION IS USED FOR THE QUATERNION

%% INPUT 
% q -> 4x1 array (quaternion)
%% OUTPUT 
% R -> 3x3 matrix (rotation matrix)
q0 = q(4); 
q1 = q(1);
q2 = q(2);
q3 = q(3);

R = [q0^2+q1^2-q2^2-q3^2 2*q1*q2+2*q0*q3 2*q1*q3-2*q0*q2;
    2*q1*q2-2*q0*q3 q0^2-q1^2+q2^2-q3^2 2*q2*q3+2*q0*q1;
    2*q1*q3+2*q0*q2 2*q2*q3-2*q0*q1 q0^2-q1^2-q2^2+q3^2];
end

== matlab function SimulinkLibrary/Performance Block /Mo/MATLAB Function ==
  data: X input; Mo output; V input
function Mo = ECI_to_ORF(X,V)

A=cross(cross(-X,V),-X);
B=norm(A);

C=cross(-X,V);
D=norm(C);

E=-X;
F=norm(X);

Mo=[A(1)/B  A(2)/B  A(3)/B;
    
    C(1)/D  C(2)/D  C(3)/D;
    
    E(1)/F  E(2)/F  E(3)/F];


end

== matlab function SimulinkLibrary/Discrete Drag in ECI/DRAG FORCE IN ORF [N]/MATLAB Function ==
  data: z input; density output
% ATMOSPHERE calculates density for altitudes from sea level
% through 1000 km using exponential interpolation.
%wwwwwwwwwwwwwwwwwwwwwwwwwwwwwwwwwwwwwwwwwwwwwwwww
%function density = atmosphere(z)
%z[km]
function density = atmosphere(z)
%...Geometric altitudes (km):
h = ...
[ 0 25 30 40 50 60 70 ...
80 90 100 110 120 130 140 ...
150 180 200 250 300 350 400 ...
450 500 600 700 800 900 1000];
%...Corresponding densities (kg/m^3) from USSA76:
r = ...
[1.225 4.008e-2 1.841e-2 3.996e-3 1.027e-3 3.097e-4 8.283e-5 ...
1.846e-5 3.416e-6 5.606e-7 9.708e-8 2.222e-8 8.152e-9 3.831e-9 ...
2.076e-9 5.194e-10 2.541e-10 6.073e-11 1.916e-11 7.014e-12 2.803e-12 ...
1.184e-12 5.215e-13 1.137e-13 3.070e-14 1.136e-14 5.759e-15 3.561e-15];
%...Scale heights (km):
H = ...
[ 7.310 6.427 6.546 7.360 8.342 7.583 6.661 ...
5.927 5.533 5.703 6.782 9.973 13.243 16.322 ...
21.652 27.974 34.934 43.342 49.755 54.513 58.019 ...
60.980 65.654 76.377 100.587 147.203 208.020];
%...Handle altitudes outside of the range:

if z > 1000
z = 1000;
elseif z < 0
z = 0;
end

i=0;  %initialize i

%...Determine the interpolation interval:
for j = 1:27
if z >= h(j) && z < h(j+1)
i = j;
end
end
if z == 1000
i = 27;
end
%...Exponential interpolation:
density = r(i)*exp(-(z - h(i))/H(i));
end %atmosphere
% %wwwwwwwwwwwwwwwwwwwwwwwwwwwwwwwwwwwwwwwwwwwwwwwww
%

== matlab function SimulinkLibrary/AeroTorque in BRF/MATLAB Function ==
  data: z input; density output
% ATMOSPHERE calculates density for altitudes from sea level
% through 1000 km using exponential interpolation.
%wwwwwwwwwwwwwwwwwwwwwwwwwwwwwwwwwwwwwwwwwwwwwwwww
%function density = atmosphere(z)
%z[km]
function density = atmosphere(z)
%...Geometric altitudes (km):
h = ...
[ 0 25 30 40 50 60 70 ...
80 90 100 110 120 130 140 ...
150 180 200 250 300 350 400 ...
450 500 600 700 800 900 1000];
%...Corresponding densities (kg/m^3) from USSA76:
r = ...
[1.225 4.008e-2 1.841e-2 3.996e-3 1.027e-3 3.097e-4 8.283e-5 ...
1.846e-5 3.416e-6 5.606e-7 9.708e-8 2.222e-8 8.152e-9 3.831e-9 ...
2.076e-9 5.194e-10 2.541e-10 6.073e-11 1.916e-11 7.014e-12 2.803e-12 ...
1.184e-12 5.215e-13 1.137e-13 3.070e-14 1.136e-14 5.759e-15 3.561e-15];
%...Scale heights (km):
H = ...
[ 7.310 6.427 6.546 7.360 8.342 7.583 6.661 ...
5.927 5.533 5.703 6.782 9.973 13.243 16.322 ...
21.652 27.974 34.934 43.342 49.755 54.513 58.019 ...
60.980 65.654 76.377 100.587 147.203 208.020];
%...Handle altitudes outside of the range:

if z > 1000
z = 1000;
elseif z < 0
z = 0;
end

i=0;  %initialize i

%...Determine the interpolation interval:
for j = 1:27
if z >= h(j) && z < h(j+1)
i = j;
end
end
if z == 1000
i = 27;
end
%...Exponential interpolation:
density = r(i)*exp(-(z - h(i))/H(i));
end %atmosphere
% %wwwwwwwwwwwwwwwwwwwwwwwwwwwwwwwwwwwwwwwwwwwwwwwww
%

== matlab function SimulinkLibrary/RWs Power Profile Check/MATLAB Function ==
  data: h_wh input; T_RWs output; Tw_4Comp input; T_lim output; T_lim_inf output
function [T_RWs,T_lim,T_lim_inf] = T_wheels(h_wh, Tw_4Comp)

% h_wh = RWs angular momentum (given by the integration of T_RWs);
% Tw_4Comp = RWs Torques without friction;

% RWs angular velocities;

omega=zeros(4,1);
omega(1)=h_wh(1)/0.000250;
omega(2)=h_wh(2)/0.000250;
omega(3)=h_wh(3)/0.000250;
omega(4)=h_wh(4)/0.000250;




T_RWs=zeros(4,1);
T_RWs(1)=Tw_4Comp(1);
T_RWs(2)=Tw_4Comp(2);
T_RWs(3)=Tw_4Comp(3);
T_RWs(4)=Tw_4Comp(4);


%% Final Comparison


   if h_wh(1) > 0
      T_max1 = 0.006-0.06*h_wh(1);
      T_min1 = -0.006;
   else
      T_max1 = 0.006;
      T_min1 = -0.006-0.06*h_wh(1);
   end

    if h_wh(2) > 0
      T_max2 = 0.006-0.06*h_wh(2);
      T_min2 = -0.006;
   else
      T_max2 = 0.006;
      T_min2 = -0.006-0.06*h_wh(2);
    end

   if h_wh(3) > 0
      T_max3 = 0.006-0.06*h_wh(3);
      T_min3 = -0.006;
   else
      T_max3 = 0.006;
      T_min3 = -0.006-0.06*h_wh(3);
   end

   if h_wh(4) > 0
      T_max4 = 0.006-0.06*h_wh(4);
      T_min4 = -0.006;
   else
      T_max4 = 0.006;
      T_min4 = -0.006-0.06*h_wh(4);
   end

   if T_RWs(1) > T_max1 
      T_RWs(1) = T_max1;
   end
   
   if T_RWs(1) < T_min1
      T_RWs(1) = T_min1;
   end

   if T_RWs(2) > T_max2 
      T_RWs(2) = T_max2;
   end
   
   if T_RWs(2) < T_min2
      T_RWs(2) = T_min2;
   end

   if T_RWs(3) > T_max3 
      T_RWs(3) = T_max3;
   end
   
   if T_RWs(3) < T_min3
      T_RWs(3) = T_min3;
   end

   if T_RWs(4) > T_max4 
      T_RWs(4) = T_max4;
   end
   
   if T_RWs(4) < T_min4
      T_RWs(4) = T_min4;
   end
   


    

%% Final Construction
T_RWs=[T_RWs(1);T_RWs(2);T_RWs(3);T_RWs(4)];
T_lim=[T_max1;T_max2;T_max3;T_max4];
T_lim_inf=[T_min1;T_min2;T_min3;T_min4];



end

== matlab function SimulinkLibrary/Magnetic Torque/Earth magnetc Field/Earth magnetic field  ==
  data: r_ECEF input; B output; nmax input; mmax input; K input; G input; H input
function B = fcn(r_ECEF, nmax, mmax, K, G, H)

R_mean = 6371.2; % Mean radius for International Geomagnetic Reference Field
e1 = [1 0 0];
e2 = [0 1 0];
e3 = [0 0 1];

A = zeros(nmax+3, mmax+3);
ctilde = zeros(nmax+3,1);
stilde = zeros(nmax+3,1);

[A, ctilde, stilde] = recursion(r_ECEF, nmax, mmax);

rho = norm(r_ECEF);
r_vers = r_ECEF'/rho;

u = r_vers(3); % argumento of latitude
B = [0 0 0];

scalar = (R_mean/rho)^2;
ttilde = G;
b1 = ttilde;
b2 = ttilde;
b3 = ttilde;
br = ttilde;
for n=1:nmax
    
   scalar = scalar*R_mean/rho;
   
   i = n+1;
    for m =0:n 
        
        j = m+1;
        
        if m <= mmax
            ttilde(i,j) = G(i,j)*ctilde(j) + H(i,j)*stilde(j);
            
            b3(i,j) =  -ttilde(i,j)*A(i,j+1);
            
            br(i,j) = ttilde(i,j)*(u*A(i,j+1) + (n+m+1)*A(i,j));
            
            B = B + scalar*K(i,j)*(b3(i,j)*e3 + br(i,j)*r_vers);
        end 
        
    if ((m > 0) && (m <= mmax))
        
        b1(i,j) = -m*A(i,j)*(G(i,j)*ctilde(j-1) + H(i,j)*stilde(j-1));
        
        b2(i,j) = -m*A(i,j)*(H(i,j)*ctilde(j-1) - G(i,j)*stilde(j-1));
        
        B = B + scalar*K(i,j)*(b1(i,j)*e1 + b2(i,j)*e2);
    end 
    end 

end
end

function [A, ctilde, stilde] = recursion(r, nmax, mmax)
A = zeros(nmax+3, mmax+3);

R_m = norm(r);
rhat = r./R_m;
u = rhat(3);

A(1,1) = 1;
A(2,1) = u;
A(2,2) = 1;

ctilde = zeros(nmax+3,1);
stilde = zeros(nmax+3,1);

ctilde(1) = 1;
ctilde(2) = rhat(1);
stilde(1) = 0;
stilde(2) = rhat(2);

for n = 2:nmax
    i = n+1;
    
    A(i,i) = prod(1:2:(2*n-1));
    A(i,i-1) = u*A(i,i);
    
    if n<=nmax
        
        ctilde(i) = ctilde(2) * ctilde(i-1) - stilde(2) * stilde(i-1);
        stilde(i)  = stilde(2) * ctilde(i-1) + ctilde(2) * stilde(i-1);
        
    end
  for m = 0:n
      
    j=m+1;
    
    if (m < (n-1)) && (m <= (mmax+1))
        
      A(i,j)=((2*n - 1)*u*A((i-1),j) - (n+m-1)*A((i-2),j))/(n-m);
      
    end

  end
end 
end

== matlab function SimulinkLibrary/Performance Block /MATLAB Function ==
  data: DCM input; roll output; pitch output; yaw output
function [roll, pitch, yaw] = calc_angles(DCM)
%321 DCM ORF->BRF;

%Angles' computation from the rotation matrix 321;
pitch=asin(-DCM(1,3));          %pitch angle (beta);
roll=atan2(DCM(2,3),DCM(3,3)); %roll angle (alpha);
yaw=atan2(DCM(1,2),DCM(1,1));  %yaw angle (gamma);

end

== matlab function SimulinkLibrary/IRF2ORF ==
  data: R_IRF input; Mo output; V_IRF input
function Mo = ECI_to_ORF(R_IRF,V_IRF)

A=cross(cross(-X,V),-X);
B=norm(A);

C=cross(-X,V);
D=norm(C);

E=-X;
F=norm(X);

Mo=[A(1)/B  A(2)/B  A(3)/B;
    
    C(1)/D  C(2)/D  C(3)/D;
    
    E(1)/F  E(2)/F  E(3)/F];


end

== matlab function SimulinkLibrary/IRF2BRF ==
  data: q input; R output
function R = R_by_q(q)

%% Description 
% This block provides the rotation matrix corresponding to the quaternion
% in input. THE SCALAR LAST CONVENTION IS USED FOR THE QUATERNION

%% INPUT 
% q -> 4x1 array (quaternion)
%% OUTPUT 
% R -> 3x3 matrix (rotation matrix)
q0 = q(4); 
q1 = q(1);
q2 = q(2);
q3 = q(3);

R = [q0^2+q1^2-q2^2-q3^2 2*q1*q2+2*q0*q3 2*q1*q3-2*q0*q2;
    2*q1*q2-2*q0*q3 q0^2-q1^2+q2^2-q3^2 2*q2*q3+2*q0*q1;
    2*q1*q3+2*q0*q2 2*q2*q3-2*q0*q1 q0^2-q1^2-q2^2+q3^2];
end

== matlab function SimulinkLibrary/Equations of motion of the spacecraft ==
  data: f input; drag input; m input; I input; h_w input; T_control input; dfdt output; T_ext input
function dfdt = SpacecraftDynamicsSimulator(f, drag, m,I,h_w, T_control, T_ext)
%#codegen

%% Copyright Università di Napoli "Federico II" - Tutti i diritti sono riservati
%
% This function calculates the spacecraft acceleration from its
% position and velocity at time t.
%----------------------------------------------------------------------
mu = 398600; %Gravitational parameter (km^3/s^2)
RE = 6378; %Earth's radius (km)

x = f(1);    %Position vector component 1st axis (km)
y = f(2);    %Position vector component 2nd axis (km)
z = f(3);    %Position vector component 3rd axis (km)

R = f(1:3)'; %Position vector (km/s)
r = norm(R); %Distance from earth's center (km)

V = f(4:6);   %Velocity vector in ECI (km/s);

% Gravitational Perturbations Coefficients

J2 = 0.00108263;
J3 = -2.33936e-3*J2;
J4 = -1.49601e-3*J2;

% Central Body Keplerian Gravity
a0 = -mu*R/r^3; %Gravitational acceleration (km/s^2)

% Gravitational perturbation acceleration
a_J2 = 3*J2*mu*RE^2/2*...
    [x*5*z^2*(x^2+y^2+z^2)^(-7/2) - x*(x^2+y^2+z^2)^(-5/2),...
    y*5*z^2*(x^2+y^2+z^2)^(-7/2) - y*(x^2+y^2+z^2)^(-5/2),...
    5*z^3*(x^2+y^2+z^2)^(-7/2) - 3*z*(x^2+y^2+z^2)^(-5/2)];

a_J3 = 5*J3*mu*RE^3/2*...
    [-3*x*z*(x^2+y^2+z^2)^(-7/2) + 7*x*z^3*(x^2+y^2+z^2)^(-9/2),...
    -3*y*z*(x^2+y^2+z^2)^(-7/2) + 7*y*z^3*(x^2+y^2+z^2)^(-9/2),...
    3/5*(x^2+y^2+z^2)^(-5/2) - 6*z^2*(x^2+y^2+z^2)^(-7/2) + 7*z^4*(x^2+y^2+z^2)^(-9/2)];
a_J4 = 15*J4*mu*RE^4/8*...
    [x*(x^2+y^2+z^2)^(-7/2) - 14*x*z^2*(x^2+y^2+z^2)^(-9/2) + 21*x*z^4*(x^2+y^2+z^2)^(-11/2),...
    y*(x^2+y^2+z^2)^(-7/2) - 14*y*z^2*(x^2+y^2+z^2)^(-9/2) + 21*y*z^4*(x^2+y^2+z^2)^(-11/2),...
    5*z*(x^2+y^2+z^2)^(-7/2) - 70/3*z^3*(x^2+y^2+z^2)^(-9/2) + 21*z^5*(x^2+y^2+z^2)^(-11/2)];

% Translational Propagation equation (i.e. translational dynamic model)
a = a0 - drag'*(1/m)*(1/1000) + a_J2 + a_J3 + a_J4; %Total acceleration (km/s^2)

%% Rotational Dynamics;

w = f(7:9);       %Angular Velocity after the integration;

p = w(1);         %Angular Velocity component ECI (1st axis)
q = w(2);         %Angular Velocity component ECI (2nd axis)
r = w(3);         %Angular Velocity component ECI (3rd axis)

J=inv(I);          %inverse inertia matrix;
h=I*w;             %angular momentum of the spacecraft;
A=cross(w,h+h_w);  %cross product;

    
w_dot=J*(T_ext-T_control-A); %% Angular velocity rate of the body in the ECI reference frame

   
%% Quaternions kynematics
q0 = f(10:13);                   %quaternion components (slide 5 of presentation lesson 2)
skew_mat = -[0 -w(3) w(2)        %Skew matrix for angular velocity quaternion multiplication (slide 5 of presentation lesson 2)  
            w(3) 0 -w(1)
           -w(2) w(1) 0];

q_dot_vec = 0.5*skew_mat*q0(1:3)+0.5*q0(4)*w;   %quaternion kinematics rate for propagation
q_dot_4 = -0.5*w'*q0(1:3);
q_dot = [q_dot_vec',q_dot_4]';                  %recollecting
%% Outputs
 
P = 2*pi*sqrt(6680^3/mu);
omegaOrb = [0;-2*pi/P;0];
dfdt = [V a w_dot' q_dot']'; %Velocity and the acceleraion returned to ode45
%ciccio_caputo =1;
end
